simulink model "Filter_2016a_tuned_on_h"  (R2016a)
settings: Solver=FixedStepDiscrete  SolverMode=SingleTasking  StartTime=0.0  StopTime=0.6  FixedStep=Ts  RelTol=1e-3
InitFcn:
  | Ts=5e-6;
  | f=50;
  | w=2*pi*f;
undefined symbols (not defined in the file): powergui, sps_lib
libraries: powerlib x27, powerlib_meascontrol x4
settings Model: Creator=Aminsystem  LastModifiedBy=Aminsystem
settings DataIOCC: SaveOutput=off  SignalLogging=off  DSMLogging=off  SaveTime=off
settings DebuggingCC: UnconnectedInputMsg=none  UnconnectedOutputMsg=none  UnconnectedLineMsg=none  SFUnexpectedBacktrackingDiag=error  SFNoUnconditionalDefaultTransitionDiag=error
settings ModelReferenceCC: EnableRefExpFcnMdlSchedulingChecks=off
settings SFSimCC: SimUseLocalCustomCode=on
settings RTWCC: Description=Generic Real-Time Target  RTWUseLocalCustomCode=on
settings GRTTargetCC: TargetLangStandard=C99 (ISO)
settings ConfigComp: CovMetricSettings=dwe  CovSaveCumulativeToWorkspaceVar=off  CovSaveSingleToWorkspaceVar=off  CovExternalEMLEnable=on

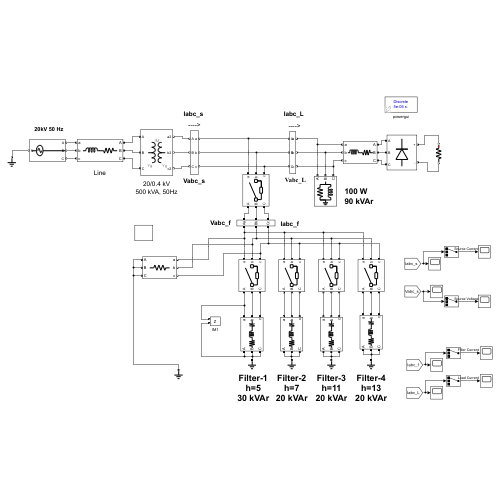
[thumbnail: Simulink's stored preview of the top-level diagram]
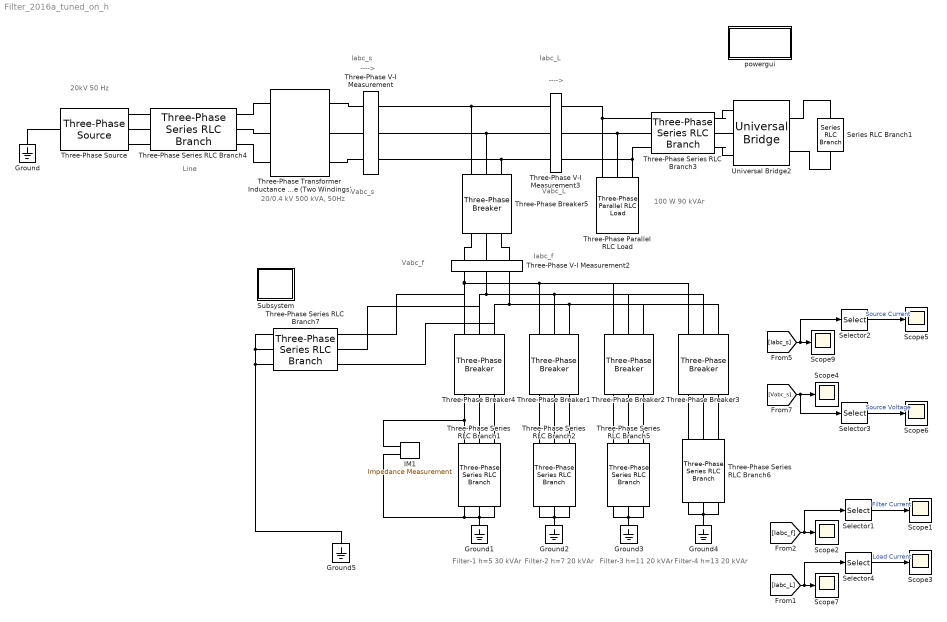
== system Filter_2016a_tuned_on_h ==
  note: Line
  note: Filter-1
      | h=5
      | 30 kVAr
  note: 100 W
      | 90 kVAr
  note: 20kV 50 Hz
  note: Iabc_L
  note: Vabc_s
  note: Iabc_s
  note: ---->
  note: ---->
  note: Vabc_L
  note: Iabc_f
  note: Vabc_f
  note: 20/0.4 kV
      | 500 kVA, 50Hz
  note: Filter-2
      | h=7
      | 20 kVAr
  note: Filter-3
      | h=11
      | 20 kVAr
  note: Filter-4
      | h=13
      | 20 kVAr
  Ground{,1..5} (6 alike) : powerlib/Elements/Ground  LConnTagsString=a
  IM1 : powerlib/Measurements/Impedance Measurement  LConnTagsString=+|-  Factor=1
  Scope{1..7,9} (8 alike) : Scope
  Selector{1..4} (4 alike) : Selector  InputPortWidth=3  IndexOptions=Index vector (dialog)  Indices=[1]  OutputSizes=1
  Series RLC Branch1 : powerlib/Elements/Series RLC Branch  LConnTagsString=__new0  RConnTagsString=__new0  BranchType=R  Resistance=400*400/180e3  Inductance=0.5e-3  SetiL0=off  InitialCurrent=0  Capacitance=1e-6  Setx0=off  InitialVoltage=0  Measurements=None
  Subsystem : Subsystem
  Three-Phase Parallel RLC Load : powerlib/Elements/Three-Phase Parallel RLC Load  LConnTagsString=A|B|C  Configuration=Y (grounded)  NominalVoltage=400  Vabc=[1e3 1e3 1e3]  Vabcp=[1e3 1e3 1e3]  NominalFrequency=50  UnbalancedPower=off  ActivePower=100  InductivePower=90e3  CapacitivePower=0  Pabc=[10e3 9e3 11e3]  QLabc=[100 90 110]  QCabc=[100 90 110]  Pabcp=[10e3 9e3 11e3]  QLabcp=[100 90 110]  QCabcp=[100 90 110]  Measurements=None  LoadType=constant Z
  Three-Phase Series RLC Branch1 : powerlib/Elements/Three-Phase Series RLC Branch  LConnTagsString=A|B|C  RConnTagsString=A|B|C  BranchType=RLC  Resistance=400*400/30e3/5/100  Inductance=400*400/30e3/5/5/w  Capacitance=30e3/(400*400*w)  Measurements=None
  Three-Phase Series RLC Branch2 : powerlib/Elements/Three-Phase Series RLC Branch  LConnTagsString=A|B|C  RConnTagsString=A|B|C  BranchType=RLC  Resistance=400*400/20e3/7/100  Inductance=400*400/20e3/7/7/w  Capacitance=20e3/(400*400*w)  Measurements=None
  Three-Phase Series RLC Branch3 : powerlib/Elements/Three-Phase Series RLC Branch  LConnTagsString=A|B|C  RConnTagsString=A|B|C  BranchType=RL  Resistance=0.1e-3  Inductance=0.1e-3  Capacitance=1e-6  Measurements=None
  Three-Phase Series RLC Branch4 : powerlib/Elements/Three-Phase Series RLC Branch  LConnTagsString=A|B|C  RConnTagsString=A|B|C  BranchType=RL  Resistance=1  Inductance=16e-3  Capacitance=1e-6  Measurements=None
  Three-Phase Series RLC Branch5 : powerlib/Elements/Three-Phase Series RLC Branch  LConnTagsString=A|B|C  RConnTagsString=A|B|C  BranchType=RLC  Resistance=400*400/20e3/11/100  Inductance=400*400/20e3/11/11/w  Capacitance=20e3/(400*400*w)  Measurements=None
  Three-Phase Series RLC Branch6 : powerlib/Elements/Three-Phase Series RLC Branch  LConnTagsString=A|B|C  RConnTagsString=A|B|C  BranchType=RLC  Resistance=400*400/20e3/13/100  Inductance=400*400/20e3/13/13/w  Capacitance=20e3/(400*400*w)  Measurements=None
  Three-Phase Series RLC Branch7 : powerlib/Elements/Three-Phase Series RLC Branch  LConnTagsString=A|B|C  RConnTagsString=A|B|C  BranchType=R  Resistance=1e5  Inductance=400*400/30e3/5/5/w  Capacitance=30e3/(400*400*w)  Measurements=None
  Three-Phase V-I Measurement : powerlib/Measurements/Three-Phase V-I Measurement  VoltageMeasurement=phase-to-ground  SetLabelV=on  LabelV=Vabc_s  Vpu=off  VpuLL=off  CurrentMeasurement=yes  SetLabelI=on  LabelI=Iabc_s  Ipu=off  Pbase=100e6  Vbase=500e3  OutputType=Complex  PhasorSimulation=off  PSBequivalent=0
  Three-Phase V-I Measurement2 : powerlib/Measurements/Three-Phase V-I Measurement  VoltageMeasurement=phase-to-ground  SetLabelV=on  LabelV=Vabc_f  Vpu=off  VpuLL=off  CurrentMeasurement=yes  SetLabelI=on  LabelI=Iabc_f  Ipu=off  Pbase=100e6  Vbase=500e3  OutputType=Complex  PhasorSimulation=off  PSBequivalent=0
  Three-Phase V-I Measurement3 : powerlib/Measurements/Three-Phase V-I Measurement  VoltageMeasurement=phase-to-ground  SetLabelV=on  LabelV=Vabc_L  Vpu=off  VpuLL=off  CurrentMeasurement=yes  SetLabelI=on  LabelI=Iabc_L  Ipu=off  Pbase=100e6  Vbase=500e3  OutputType=Complex  PhasorSimulation=off  PSBequivalent=0
  Three-Phase Breaker1 : powerlib/Elements/Three-Phase Breaker  InitialState=open  SwitchA=on  SwitchB=on  SwitchC=on  SwitchTimes=[0.25]  External=off  BreakerResistance=0.001  SnubberResistance=1e7  SnubberCapacitance=inf  Measurements=None
  Three-Phase Breaker2 : powerlib/Elements/Three-Phase Breaker  InitialState=open  SwitchA=on  SwitchB=on  SwitchC=on  SwitchTimes=[0.3]  External=off  BreakerResistance=0.001  SnubberResistance=1e7  SnubberCapacitance=inf  Measurements=None
  Three-Phase Breaker3 : powerlib/Elements/Three-Phase Breaker  InitialState=open  SwitchA=on  SwitchB=on  SwitchC=on  SwitchTimes=[0.35]  External=off  BreakerResistance=0.001  SnubberResistance=1e7  SnubberCapacitance=inf  Measurements=None
  Three-Phase Breaker4 : powerlib/Elements/Three-Phase Breaker  InitialState=open  SwitchA=on  SwitchB=on  SwitchC=on  SwitchTimes=[0.2]  External=off  BreakerResistance=0.001  SnubberResistance=1e7  SnubberCapacitance=inf  Measurements=None
  Three-Phase Breaker5 : powerlib/Elements/Three-Phase Breaker  InitialState=open  SwitchA=on  SwitchB=on  SwitchC=on  SwitchTimes=[0.2]  External=off  BreakerResistance=0.001  SnubberResistance=1e7  SnubberCapacitance=inf  Measurements=None
  Three-Phase Source : powerlib/Electrical Sources/Three-Phase Source  InternalConnection=Yn  VoltagePhases=off  Voltage=20e3  PhaseAngle=0  Voltage_phases=[25e3 25e3 25e3]/sqrt(3)  PhaseAngles_phases=[0 -120 +120]  Frequency=50  NonIdealSource=off  SpecifyImpedance=off  Resistance=0.8929  Inductance=16.58e-3  ShortCircuitLevel=100e6  BaseVoltage=20e3  XRratio=10  BusType=swing  Pref=10e3  Qref=0  Prefabc=[10e3, 10e3, 10e3]  Qrefabc=[0, 0, 0]  Qmin=-inf  Qmax=inf
  Three-Phase Transformer Inductance Matrix Type (Two Windings) : powerlib/Elements/Three-Phase Transformer Inductance Matrix Type (Two Windings)  CoreType=Three single-phase cores  Winding1Connection=Yg  Winding2Connection=Yg  AutoTransformer=off  Measurements=None  NominalPower=[500e3, 50]  VLLnom=[20e3, 400]  WindingResistances=[0.01, 0.01]  NoLoadIexcPos=2  NoLoadPlossPos=250  ShortCircuitReactancePos=0.06  ShortCircuitReactancePosAuto=0.06  NoLoadIexcZero=100  NoLoadPlossZero=1500  ShortCircuitReactanceZero=0.03  ShortCircuitReactanceZeroAuto=0.03
  Universal Bridge2 : powerlib/Power Electronics/Universal Bridge  Arms=3  SnubberResistance=1e5  SnubberCapacitance=inf  Device=Diodes  Ron=1e-3  Lon=0  ForwardVoltages="[  0  0  ]"  ForwardVoltage=0  GTOparameters=[ 10e-6 , 20e-6 ]  IGBTparameters=[ 1e-6 , 2e-6 ]  Measurements=None  Measurements_2=None  converterType=Rectifier
  powergui : Subsystem  Priority=1  AncestorBlock=sps_lib/powergui  DialogController=POWERSYS.PowerSysDialog  InitFcn=powergui( 'InitFcn_Callback' , gcb , 0 , [ ] );  mask(PSB option menu block){SimulationMode=Discrete, SampleTime=Ts, frequency=60, Iterations=50, frequencyindice=0, Pbase=100e6, ErrMax=1e-4, UnitsV=kV, UnitsW=MW, buscounter=0, FunctionMessages=off, echomessages=off, EnableUseOfTLC=off, CurrentSourceSwitches=off, DisableSnubberDevices=off, DisableRonSwitches=off, DisableVfSwitches=off, DisplayEquations=off, AutomaticDiscreteSolvers=off, SolverType=Tustin, Interpol=off, ExternalGateDelay=off, methode=off, Ts=100, x0status=blocks, SPID=on, SwTol=0, HookPort=off, NonlinearTolerance=1e-4, nMaxIteration=100, ContinueOnMaxIteration=off, RestoreLinks=warning, ResistiveCurrentMeasurement=off, Frange=[0:2:500], Ylog=off, Xlog=on, ShowGrid=off, save=off, variable=ZData, structure=Iabc_s, ZoomFFT=off, StartTime=1.6, cycles=20, DisplayStyle=1, fundamental=50, FreqAxis=on, MaxFrequency=50*20, frequencyindicesteady=1, RmsSteady=1, display=off}
      mask prompts: SimulationMode "Simulation type:"; SampleTime "Sample time (s):"; frequency "Frequency (Hz):"; Iterations "Max iterations"; frequencyindice "Frequency (Hz)"; Pbase "Base power (VA)"; ErrMax "PQ tolerance (pu)"; UnitsV "Voltage units"; UnitsW "Power units"; buscounter "Load flow bus counter"; FunctionMessages "Disable Specialized Power Systems warnings"; echomessages "Display Specialized Power Systems compilation messages"; EnableUseOfTLC "Use TLC file when in Accelerator Simulation Mode and for code generation"; CurrentSourceSwitches "Disable ideal switching"; DisableSnubberDevices "Disable snubbers in switching devices"; DisableRonSwitches "Disable Ron resistances in switching devices"; DisableVfSwitches "Disable forward voltages in switching devices"; DisplayEquations "Display circuit differential equations"; AutomaticDiscreteSolvers "Automatically handle Discrete solver and Advanced tab solver settings of blocks"; SolverType "Discrete solver"; Interpol "Interpolate switching events"; ExternalGateDelay "Use time-stamped gate signals"; methode "Store switching topologies"; Ts "Buffer size (MBytes):"; x0status "Start simulation with initial electrical states from:"; SPID "Use ideal switching devices"; SwTol "Switch tolerance"; HookPort "Allow multiple powergui blocks"; NonlinearTolerance "Solver tolerance"; nMaxIteration "Maximum number of iterations"; ContinueOnMaxIteration "Continue Simulation if maximum number of iterations is reached"; RestoreLinks "Restore disabled links of Simscape Power Systems ST blocks:"; ResistiveCurrentMeasurement "Use non ideal current measurement blocks (1e-4Ohm internal resistance)"; Frange "Frequency Range"; Ylog "Log impedance"; Xlog "log Frequency"; ShowGrid "grid"; save "Save Data To Workspace"; variable "Variable Name"; structure "Structure Name (PSBFFTSCOPE)"; ZoomFFT "ZoomFFT (PSBFFTSCOPE)"; StartTime "Start Time (PSBFFTSCOPE)"; cycles "Cycles (PSBFFTSCOPE)"; DisplayStyle "Display style (PSBFFTSCOPE)"; fundamental "Fundamental (PSBFFTSCOPE)"; FreqAxis "Frequency Axis (PSBFFTSCOPE)"; MaxFrequency "Max Frequency (PSBFFTSCOPE)"; frequencyindicesteady "Frequency indice (STEADYSTATE)"; RmsSteady "RMS display (STEADYSTATE)"; display "Display Results"
      mask help: Set simulation type, simulation parameters, and preferences.
      mask init:
      | dispMessage = '';
      | dispMessage = powergui('MaskInitialization',gcb,SimulationMode,SampleTime);
      settings: PreSaveFcn=powergui( 'PreSaveFcn_Callback' , gcb , [ ] , [ ] );  OpenFcn=sps_rtmsupport('OpenFcn',gcbh)
      mask Help: helpview(psbhelp)
      mask TypeOptions SimulationMode: Continuous | Discrete | Phasor | Discrete phasor
      mask Callback SimulationMode: powergui('SimulationType',[],[],gcb);
      mask TypeOptions UnitsV: V | kV
      mask TypeOptions UnitsW: W | kW | MW
      mask Callback CurrentSourceSwitches: powergui('SimulationType',[],[],gcb);
      mask Callback AutomaticDiscreteSolvers: powergui('SimulationType',[],[],gcb);
      mask TypeOptions SolverType: Tustin/Backward Euler (TBE) | Tustin | Backward Euler
      mask Callback SolverType: powergui('SimulationType',[],[],gcb);
      mask Callback Interpol: powergui('SimulationType',[],[],gcb);
      mask Callback ExternalGateDelay: powergui('SimulationType',[],[],gcb);
      mask Callback methode: powergui('SimulationType',[],[],gcb);
      mask TypeOptions x0status: blocks | steady | zero
      mask TypeOptions RestoreLinks: yes | warning | no
      mask Callback display: sps_rtmsupport('parametereditingmodes',gcbh) % Will be executed last in parameter callbacks to ensure mask enable consistency
      mask DialogControl AutoSolverNote Prompt: The Simulation type parameter is governed by Simulink. To access the Powergui solver settings, unselect auto (Automatic solver selection) solver in the Simulink solver options.
      mask DialogControl StateAnalyzer Prompt: Measurements and States Analyzer
      mask DialogControl StateAnalyzer Callback: powerStates(bdroot(gcb))
      mask DialogControl LineParameterCalculator Prompt: Line Parameter Calculator
      mask DialogControl LineParameterCalculator Callback:
      | close_system(gcb)
      | powerLineParameters
      mask DialogControl CableParameterCalculator Prompt: Cable Parameter Calculator
      mask DialogControl CableParameterCalculator Callback:
      | close_system(gcb)
      | powerCableParameters
      mask DialogControl LineDecoupler Prompt: Line Decoupler
      mask DialogControl LineDecoupler Tooltip: Click to replace selected Distributed Parameters Line blocks with Decoupling Line blocks
      mask DialogControl LineDecoupler Callback:
      | close_system(gcb);
      | DecouplingLineReplace(gcs)
      mask DialogControl LoadFlowAnalyzer Prompt: Load Flow Analyzer
      mask DialogControl LoadFlowAnalyzer Callback:
      | close_system(gcb)
      | powerLoadFlow
      mask DialogControl LoadFlowParameters Prompt: Load Flow Parameters
      mask DialogControl ImpedanceCalculator Prompt: Impedance Calculator
      mask DialogControl ImpedanceCalculator Callback:
      | close_system(gcb);
      | powerImpedance(bdroot(gcs));
      mask DialogControl FFTAnalyzer Prompt: FFT Analyzer
      mask DialogControl FFTAnalyzer Callback:
      | close_system(gcb)
      | power_fftscope(bdroot(gcb),gcb)
      mask DialogControl LinearSystemAnalyzer Prompt: Linear System Analyzer
      mask DialogControl LinearSystemAnalyzer Callback:
      | close_system(gcb)
      | power_ltiview(bdroot(gcb))
      mask DialogControl HysteresisDesigner Prompt: Hysteresis Designer
      mask DialogControl HysteresisDesigner Callback:
      | close_system(gcb)
      | powerHysteresis('hysteresis.mat')
      mask DialogControl BlockCustomizer Prompt: Block Customizer
      mask DialogControl BlockCustomizer Callback:
      | close_system(gcb);
      | power_customize;
      mask DialogControl ReportGenerator Prompt: Report Generator
      mask DialogControl ReportGenerator Callback:
      | close_system(gcb)
      | power_report(bdroot(gcb))
      mask DialogControl obsolete Prompt: ...
      mask DialogControl MachineInitialization Prompt: Machine Initialization
      mask DialogControl MachineInitialization Callback:
      | close_system(gcb)
      | powericon('machineInitTool',bdroot(gcb),gcb)
      mask DialogControl Solver Prompt: Solver
      mask DialogControl SolverDetails Prompt: Solver details for nonlinear elements
      mask Display: color('blue'),disp(dispMessage)
  wires:
  [Iabc_s] -> Selector2/1, Scope9/1
  Selector2/1 -> Scope5/1  "Source Current"
  [Vabc_s] -> Scope4/1, Selector3/1
  Selector3/1 -> Scope6/1  "Source Voltage"
  Selector1/1 -> Scope1/1  "Filter Current"
  [Iabc_f] -> Scope2/1, Selector1/1
  [Iabc_L] -> Selector4/1, Scope7/1
  Selector4/1 -> Scope3/1  "Load Current"
  connections:
  Three-Phase Series RLC Branch3/RConn2 -- Three-Phase Parallel RLC Load/LConn2 -- Three-Phase V-I Measurement3/RConn2
  Three-Phase Breaker5/LConn1 -- Three-Phase V-I Measurement2/RConn1
  Three-Phase V-I Measurement3/RConn3 -- Three-Phase Parallel RLC Load/LConn3 -- Three-Phase Series RLC Branch3/RConn3
  Three-Phase Series RLC Branch3/RConn1 -- Three-Phase Parallel RLC Load/LConn1 -- Three-Phase V-I Measurement3/RConn1
  Three-Phase Breaker5/LConn2 -- Three-Phase V-I Measurement2/RConn2
  Three-Phase V-I Measurement/RConn3 -- Three-Phase Breaker5/RConn3 -- Three-Phase V-I Measurement3/LConn3
  Ground/LConn1 -- Three-Phase Source/LConn1
  Three-Phase Breaker5/LConn3 -- Three-Phase V-I Measurement2/RConn3
  Three-Phase V-I Measurement/RConn1 -- Three-Phase Breaker5/RConn1 -- Three-Phase V-I Measurement3/LConn1
  Three-Phase V-I Measurement/RConn2 -- Three-Phase Breaker5/RConn2 -- Three-Phase V-I Measurement3/LConn2
  Three-Phase Series RLC Branch1/LConn1 -- Ground1/LConn1 -- Three-Phase Series RLC Branch1/LConn2 -- Three-Phase Series RLC Branch1/LConn3 -- IM1/LConn2
  Three-Phase Breaker2/RConn2 -- Three-Phase Breaker3/RConn2 -- Three-Phase Breaker1/RConn2 -- Three-Phase Series RLC Branch7/RConn2 -- Three-Phase Breaker4/RConn2 -- Three-Phase V-I Measurement2/LConn2
  Three-Phase V-I Measurement2/LConn1 -- Three-Phase Series RLC Branch7/RConn1 -- Three-Phase Breaker4/RConn1 -- Three-Phase Breaker3/RConn1 -- Three-Phase Breaker2/RConn1 -- Three-Phase Breaker1/RConn1
  Three-Phase Breaker3/RConn3 -- Three-Phase Breaker2/RConn3 -- Three-Phase Breaker1/RConn3 -- Three-Phase Series RLC Branch7/RConn3 -- Three-Phase Breaker4/RConn3 -- Three-Phase V-I Measurement2/LConn3
  Three-Phase Series RLC Branch4/RConn1 -- Three-Phase Source/RConn1
  Three-Phase Series RLC Branch4/RConn3 -- Three-Phase Source/RConn3
  Three-Phase Series RLC Branch4/RConn2 -- Three-Phase Source/RConn2
  Three-Phase Transformer Inductance Matrix Type (Two Windings)/LConn2 -- Three-Phase Series RLC Branch4/LConn2
  Three-Phase Transformer Inductance Matrix Type (Two Windings)/LConn1 -- Three-Phase Series RLC Branch4/LConn1
  Three-Phase Transformer Inductance Matrix Type (Two Windings)/LConn3 -- Three-Phase Series RLC Branch4/LConn3
  Ground3/LConn1 -- Three-Phase Series RLC Branch5/LConn2 -- Three-Phase Series RLC Branch5/LConn3 -- Three-Phase Series RLC Branch5/LConn1
  Ground4/LConn1 -- Three-Phase Series RLC Branch6/LConn2 -- Three-Phase Series RLC Branch6/LConn1 -- Three-Phase Series RLC Branch6/LConn3
  Three-Phase Transformer Inductance Matrix Type (Two Windings)/RConn1 -- Three-Phase V-I Measurement/LConn1
  Three-Phase Transformer Inductance Matrix Type (Two Windings)/RConn2 -- Three-Phase V-I Measurement/LConn2
  Three-Phase Transformer Inductance Matrix Type (Two Windings)/RConn3 -- Three-Phase V-I Measurement/LConn3
  Ground2/LConn1 -- Three-Phase Series RLC Branch2/LConn1 -- Three-Phase Series RLC Branch2/LConn3 -- Three-Phase Series RLC Branch2/LConn2
  Three-Phase Series RLC Branch2/RConn1 -- Three-Phase Breaker1/LConn1
  Three-Phase Series RLC Branch2/RConn2 -- Three-Phase Breaker1/LConn2
  Three-Phase Series RLC Branch2/RConn3 -- Three-Phase Breaker1/LConn3
  Three-Phase Breaker2/LConn1 -- Three-Phase Series RLC Branch5/RConn1
  Three-Phase Breaker2/LConn2 -- Three-Phase Series RLC Branch5/RConn2
  Three-Phase Breaker2/LConn3 -- Three-Phase Series RLC Branch5/RConn3
  Three-Phase Breaker3/LConn1 -- Three-Phase Series RLC Branch6/RConn1
  Three-Phase Breaker3/LConn2 -- Three-Phase Series RLC Branch6/RConn2
  Three-Phase Breaker3/LConn3 -- Three-Phase Series RLC Branch6/RConn3
  Three-Phase Breaker4/LConn1 -- IM1/LConn1 -- Three-Phase Series RLC Branch1/RConn1
  Three-Phase Breaker4/LConn2 -- Three-Phase Series RLC Branch1/RConn2
  Three-Phase Breaker4/LConn3 -- Three-Phase Series RLC Branch1/RConn3
  Universal Bridge2/RConn1 -- Series RLC Branch1/LConn1
  Series RLC Branch1/RConn1 -- Universal Bridge2/RConn2
  Three-Phase Series RLC Branch3/LConn2 -- Universal Bridge2/LConn2
  Three-Phase Series RLC Branch3/LConn1 -- Universal Bridge2/LConn1
  Three-Phase Series RLC Branch3/LConn3 -- Universal Bridge2/LConn3
  Three-Phase Series RLC Branch7/LConn1 -- Three-Phase Series RLC Branch7/LConn2 -- Three-Phase Series RLC Branch7/LConn3 -- Ground5/LConn1

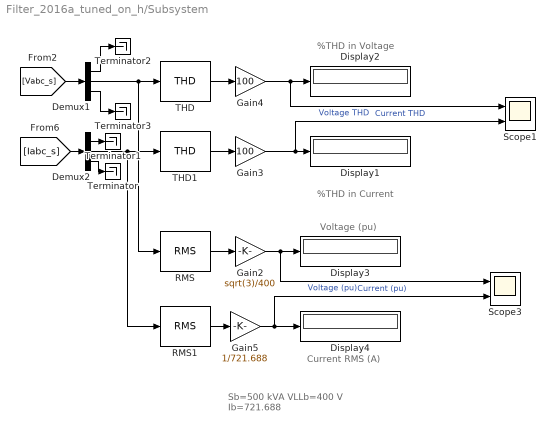
== system Filter_2016a_tuned_on_h/Subsystem ==
  note: Sb=500 kVA
      | VLLb=400 V
      | Ib=721.688
  note: %THD in Current
  note: %THD in Voltage
  note: Voltage (pu)
  note: Current RMS (A)
  Demux1 : Demux  Outputs=3
  Demux2 : Demux  Outputs=3
  Display{1..4} (4 alike) : Display
  Gain2 : Gain  Gain=sqrt(3)/400
  Gain3 : Gain  Gain=100
  Gain4 : Gain  Gain=100
  Gain5 : Gain  Gain=1/721.688
  RMS : powerlib_meascontrol/Measurements/RMS  TrueRMS=on  Freq=50  RMSInit=230  Ts=Ts
  RMS1 : powerlib_meascontrol/Measurements/RMS  TrueRMS=on  Freq=50  RMSInit=0  Ts=Ts
  Scope1 : Scope  NumInputPorts=2
  Scope3 : Scope  NumInputPorts=2
  THD : powerlib_meascontrol/Measurements/THD  Freq=50  Ts=Ts
  THD1 : powerlib_meascontrol/Measurements/THD  Freq=50  Ts=Ts
  Terminator{,1..3} (4 alike) : Terminator
  wires:
  Demux1/2 -> RMS/1, THD/1
  [Iabc_s] -> Demux2/1
  THD/1 -> Gain4/1
  Gain3/1 -> Scope1/2, Display1/1  "Current THD"
  THD1/1 -> Gain3/1
  Demux2/2 -> RMS1/1, THD1/1
  [Vabc_s] -> Demux1/1
  Gain5/1 -> Scope3/2, Display4/1  "Current (pu)"
  Gain4/1 -> Scope1/1, Display2/1  "Voltage THD"
  RMS/1 -> Gain2/1
  RMS1/1 -> Gain5/1
  Gain2/1 -> Scope3/1, Display3/1  "Voltage (pu)"
  Demux2/3 -> Terminator/1
  Demux2/1 -> Terminator1/1
  Demux1/1 -> Terminator2/1
  Demux1/3 -> Terminator3/1

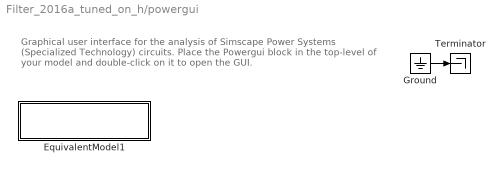
== system Filter_2016a_tuned_on_h/powergui ==
  note: Graphical user interface for the analysis of
      | Simscape Power Systems (Specialized Technology) circuits.
      | Place the Powergui block in the top-level of your model and double-click
      | on it to open the GUI.
  EquivalentModel1 : Subsystem
      mask init:
      | S  = GetDataForEquivalentModel('Discrete',gcbh);
      mask Display:
      | color('red')
      | disp('EQUIVALENT CIRCUIT\nDiscrete')
  Ground : Ground
  Terminator : Terminator
  wires:
  Ground/1 -> Terminator/1

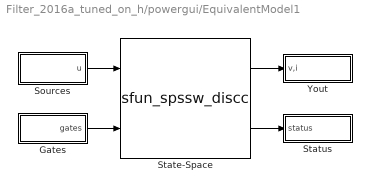
== system Filter_2016a_tuned_on_h/powergui/EquivalentModel1 ==
  Gates : Subsystem
  Sources : Subsystem
  State-Space : S-Function  FunctionName=sfun_spssw_discc  Parameters=S.Ts,S.A, S.B, S.C, S.D, S.x0, S.EnableUseOfTLC,S.SwitchResistance ,S.SwitchType, S.SwitchGateInitialValue, S.OutputsToResetToZero, S.TBEON,S.SaveMatrices,S.BufferSize  SFunctionDeploymentMode=off  EnableBusSupport=off
  Status : Subsystem
  Yout : Subsystem
  wires:
  Gates/1(gates) -> State-Space/2
  Sources/1(u) -> State-Space/1
  State-Space/2 -> Status/1(status)
  State-Space/1 -> Yout/1(v,i)

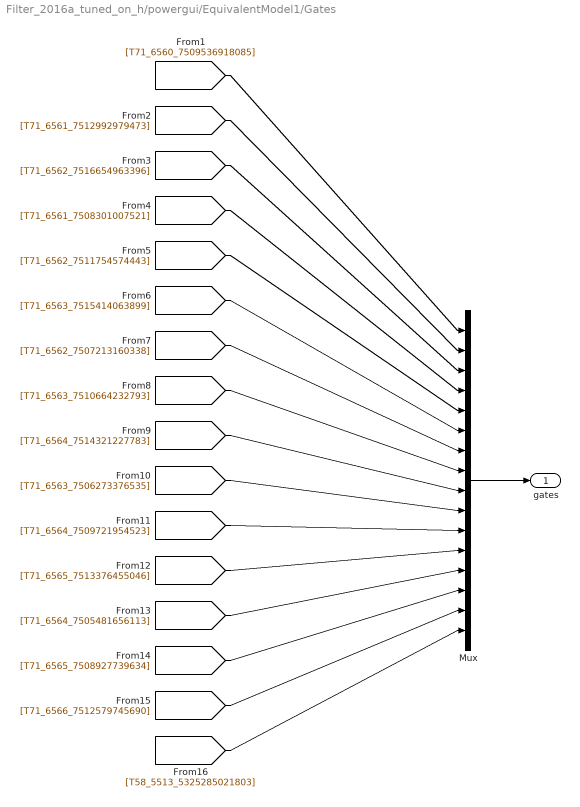
== system Filter_2016a_tuned_on_h/powergui/EquivalentModel1/Gates ==
  Mux : Mux  Inputs=[1 1 1 1 1 1 1 1 1 1 1 1 1 1 1 6]
  gates : Outport
  wires:
  Mux/1 -> gates/1
  [T71_6560_7509536918085] -> Mux/1
  [T71_6561_7512992979473] -> Mux/2
  [T71_6562_7516654963396] -> Mux/3
  [T71_6561_7508301007521] -> Mux/4
  [T71_6562_7511754574443] -> Mux/5
  [T71_6563_7515414063899] -> Mux/6
  [T71_6562_7507213160338] -> Mux/7
  [T71_6563_7510664232793] -> Mux/8
  [T71_6564_7514321227783] -> Mux/9
  [T71_6563_7506273376535] -> Mux/10
  [T71_6564_7509721954523] -> Mux/11
  [T71_6565_7513376455046] -> Mux/12
  [T71_6564_7505481656113] -> Mux/13
  [T71_6565_7508927739634] -> Mux/14
  [T71_6566_7512579745690] -> Mux/15
  [T58_5513_5325285021803] -> Mux/16

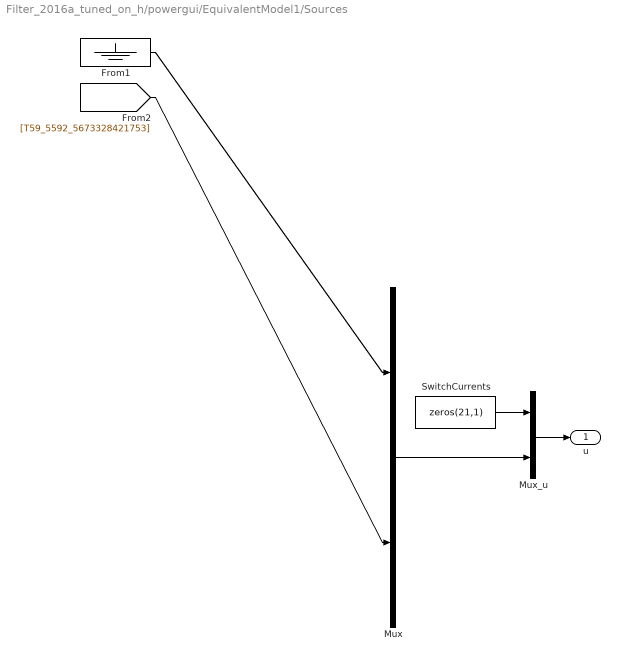
== system Filter_2016a_tuned_on_h/powergui/EquivalentModel1/Sources ==
  From1 : Ground
  Mux : Mux  Inputs=[1 3]
  Mux_u : Mux  Inputs=[21 4]
  SwitchCurrents : Constant  Value=zeros(21,1)
  u : Outport
  wires:
  Mux_u/1 -> u/1
  SwitchCurrents/1 -> Mux_u/1
  Mux/1 -> Mux_u/2
  From1/1 -> Mux/1
  [T59_5592_5673328421753] -> Mux/2

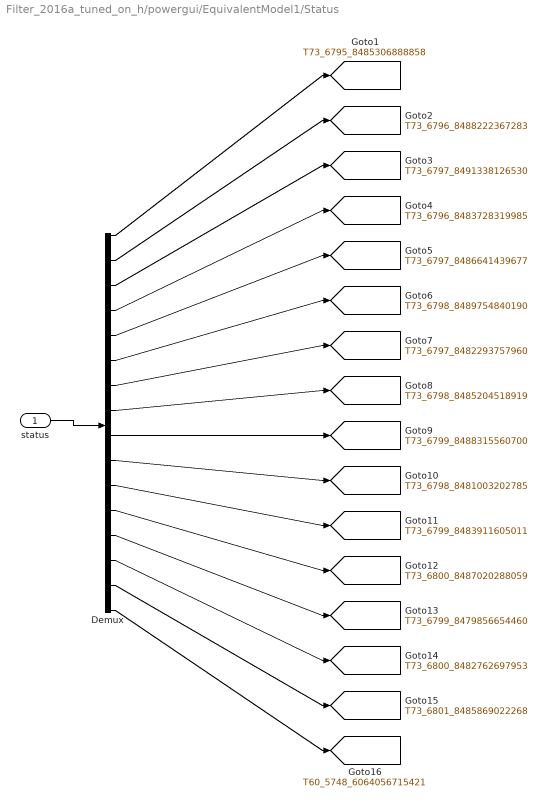
== system Filter_2016a_tuned_on_h/powergui/EquivalentModel1/Status ==
  status : Inport
  Demux : Demux  Outputs=[1 1 1 1 1 1 1 1 1 1 1 1 1 1 1 6]
  tag scope: T60_5748_6064056715421=global, T73_6795_8485306888858=global, T73_6796_8483728319985=global, T73_6796_8488222367283=global, T73_6797_8482293757960=global, T73_6797_8486641439677=global, T73_6797_8491338126530=global, T73_6798_8481003202785=global, T73_6798_8485204518919=global, T73_6798_8489754840190=global, T73_6799_8479856654460=global, T73_6799_8483911605011=global, T73_6799_8488315560700=global, T73_6800_8482762697953=global, T73_6800_8487020288059=global, T73_6801_8485869022268=global
  wires:
  status/1 -> Demux/1
  Demux/1 -> [T73_6795_8485306888858]
  Demux/2 -> [T73_6796_8488222367283]
  Demux/3 -> [T73_6797_8491338126530]
  Demux/4 -> [T73_6796_8483728319985]
  Demux/5 -> [T73_6797_8486641439677]
  Demux/6 -> [T73_6798_8489754840190]
  Demux/7 -> [T73_6797_8482293757960]
  Demux/8 -> [T73_6798_8485204518919]
  Demux/9 -> [T73_6799_8488315560700]
  Demux/10 -> [T73_6798_8481003202785]
  Demux/11 -> [T73_6799_8483911605011]
  Demux/12 -> [T73_6800_8487020288059]
  Demux/13 -> [T73_6799_8479856654460]
  Demux/14 -> [T73_6800_8482762697953]
  Demux/15 -> [T73_6801_8485869022268]
  Demux/16 -> [T60_5748_6064056715421]

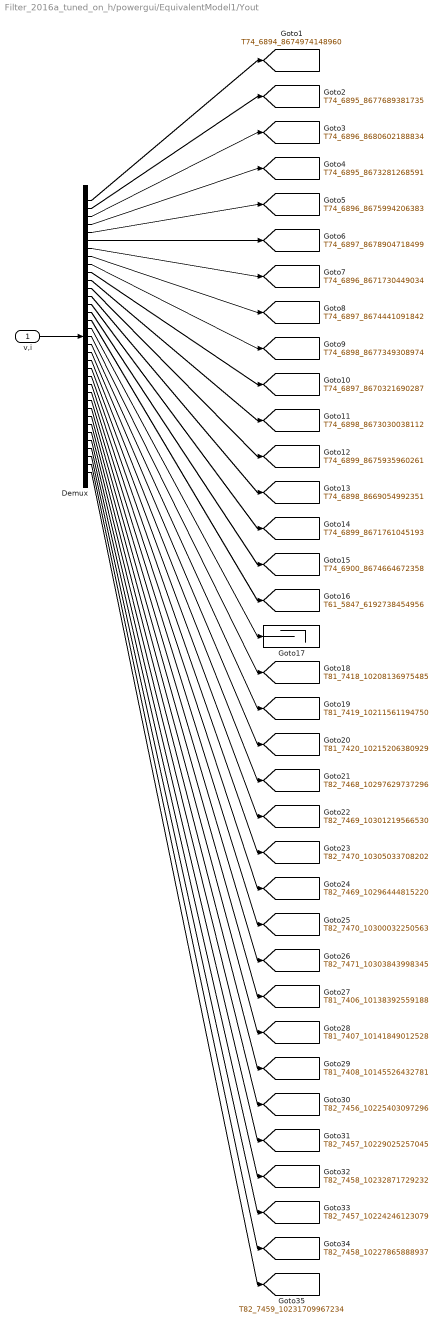
== system Filter_2016a_tuned_on_h/powergui/EquivalentModel1/Yout ==
  v,i : Inport
  Demux : Demux  Outputs=[1 1 1 1 1 1 1 1 1 1 1 1 1 1 1 6 1 1 1 1 1 1 1 1 1 1 1 1 1 1 1 1 1 1 1]
  Goto17 : Terminator
  tag scope: T61_5847_6192738454956=global, T74_6894_8674974148960=global, T74_6895_8673281268591=global, T74_6895_8677689381735=global, T74_6896_8671730449034=global, T74_6896_8675994206383=global, T74_6896_8680602188834=global, T74_6897_8670321690287=global, T74_6897_8674441091842=global, T74_6897_8678904718499=global, T74_6898_8669054992351=global, T74_6898_8673030038112=global, T74_6898_8677349308974=global, T74_6899_8671761045193=global, T74_6899_8675935960261=global, T74_6900_8674664672358=global, T81_7406_10138392559188=global, T81_7407_10141849012528=global, T81_7408_10145526432781=global, T81_7418_10208136975485=global, T81_7419_10211561194750=global, T81_7420_10215206380929=global, T82_7456_10225403097296=global, T82_7457_10224246123079=global, T82_7457_10229025257045=global, T82_7458_10227865888937=global, T82_7458_10232871729232=global, T82_7459_10231709967234=global, T82_7468_10297629737296=global, T82_7469_10296444815220=global, T82_7469_10301219566530=global, T82_7470_10300032250563=global, T82_7470_10305033708202=global, T82_7471_10303843998345=global
  wires:
  v,i/1 -> Demux/1
  Demux/1 -> [T74_6894_8674974148960]
  Demux/2 -> [T74_6895_8677689381735]
  Demux/3 -> [T74_6896_8680602188834]
  Demux/4 -> [T74_6895_8673281268591]
  Demux/5 -> [T74_6896_8675994206383]
  Demux/6 -> [T74_6897_8678904718499]
  Demux/7 -> [T74_6896_8671730449034]
  Demux/8 -> [T74_6897_8674441091842]
  Demux/9 -> [T74_6898_8677349308974]
  Demux/10 -> [T74_6897_8670321690287]
  Demux/11 -> [T74_6898_8673030038112]
  Demux/12 -> [T74_6899_8675935960261]
  Demux/13 -> [T74_6898_8669054992351]
  Demux/14 -> [T74_6899_8671761045193]
  Demux/15 -> [T74_6900_8674664672358]
  Demux/16 -> [T61_5847_6192738454956]
  Demux/17 -> Goto17/1
  Demux/18 -> [T81_7418_10208136975485]
  Demux/19 -> [T81_7419_10211561194750]
  Demux/20 -> [T81_7420_10215206380929]
  Demux/21 -> [T82_7468_10297629737296]
  Demux/22 -> [T82_7469_10301219566530]
  Demux/23 -> [T82_7470_10305033708202]
  Demux/24 -> [T82_7469_10296444815220]
  Demux/25 -> [T82_7470_10300032250563]
  Demux/26 -> [T82_7471_10303843998345]
  Demux/27 -> [T81_7406_10138392559188]
  Demux/28 -> [T81_7407_10141849012528]
  Demux/29 -> [T81_7408_10145526432781]
  Demux/30 -> [T82_7456_10225403097296]
  Demux/31 -> [T82_7457_10229025257045]
  Demux/32 -> [T82_7458_10232871729232]
  Demux/33 -> [T82_7457_10224246123079]
  Demux/34 -> [T82_7458_10227865888937]
  Demux/35 -> [T82_7459_10231709967234]
